simulink model "DAS"  (R2012b)
settings: Solver=FixedStepDiscrete  StartTime=0.0  StopTime=inf  FixedStep=0.1  RelTol=1e-3
PreLoadFcn:
  | if exist('tl_preloadfcn','file'), tl_preloadfcn(gcs,101); end
PostLoadFcn:
  | if exist('tl_postloadfcn','file'), tl_postloadfcn(gcs,101); end
InitFcn:
  | if exist('tlds_init','file'), tlds_init(gcs); end
StartFcn:
  | if exist('tlds_start','file'), tlds_start(gcs); end
StopFcn:
  | if exist('tlds_stop','file'), tlds_stop(gcs); end
undefined symbols (not defined in the file): A, B, C, Dd, DEMO_FAS_Accusti_Threshold_Time, DEMO_FAS_BrakeBooster_Threshold, DEMO_FAS_CC_DELTA, DEMO_FAS_CC_Lvl2_Round, DEMO_FAS_CC_Min_Value, DEMO_FAS_Distance_Treshold_Far, DEMO_FAS_Distance_Treshold_Med, DEMO_FAS_Distance_Treshold_Near, DEMO_FAS_Distronic, DEMO_FAS_Emerg_Brake_Force1, DEMO_FAS_Emerg_Brake_Force2, DEMO_FAS_Emerg_Brake_Time1, DEMO_FAS_Emerg_Brake_Time2, DEMO_FAS_EmergencyBrake, DEMO_FAS_FollowToStop, DEMO_FAS_Limiter, DEMO_FAS_Limiter_DELTA, DEMO_FAS_Neg_Max_ms, DEMO_FAS_Opti_Threshold_Time, DEMO_FAS_Repeater, DEMO_FAS_Repeater_Time, DEMO_FAS_Signdetection, DEMO_FAS_Tempomat
(part 2 of 11)

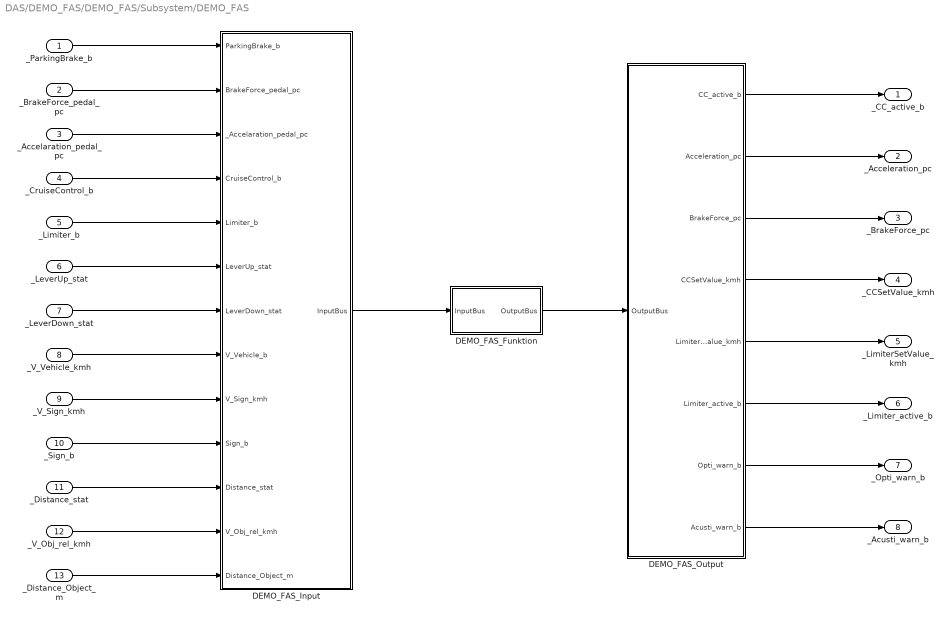
== system DAS/DEMO_FAS/DEMO_FAS/Subsystem/DEMO_FAS ==
  _ParkingBrake_b : Inport  PortDimensions=1  mask(TL_Inport){data={'output',{'variable','DEMO_FAS/i/Components/ParkingBrake_b'},'date',735342.43720311346}}
      settings: DeleteFcn=if exist('delete_tlblock','file')==2,delete_tlblock(gcbh);end  OpenFcn=if exist('tl_open_blockdlg','file')==2,tl_open_blockdlg(gcbh);else,open_system(gcbh,'parameter');end
      settings: CopyFcn=|
      | if exist('tl_reset_reviewflag','file')==2
      |     tl_reset_reviewflag(gcbh);
      | end
      | if exist('tl_check_ports','file')
      |     tl_check_ports(gcbh);
      | end
      settings: NameChangeFcn=|
      | if exist('rename_tlblock','file')==2,rename_tlblock(gcbh);end
      | if exist('tl_check_ports','file'), tl_check_ports(gcbh); end
      mask Help: eval(['if exist(''tl_online_help'',''file'') == 2, tl_online_help(''Topic'',''TL_Inport''),else, web([''jar:file:///'',matlabroot,''/help/toolbox/simulink/help.jar!/slref/' lower(get_param(gcbh,'Blocktype')) '.html''], ''-helpbrowser''),end'])
      mask Display: plot([0.2 0.35 NaN 0.65 0.8],[0 1 NaN 0 1]);
  _BrakeForce_pedal_pc : Inport  Port=2  PortDimensions=1  mask(TL_Inport){data={'output',{'variable','DEMO_FAS/i/Components/BrakeForce_pedal_pc'},'date',735342.4371075232}}
      settings: DeleteFcn=if exist('delete_tlblock','file')==2,delete_tlblock(gcbh);end  OpenFcn=if exist('tl_open_blockdlg','file')==2,tl_open_blockdlg(gcbh);else,open_system(gcbh,'parameter');end
      settings: CopyFcn=|
      | if exist('tl_reset_reviewflag','file')==2
      |     tl_reset_reviewflag(gcbh);
      | end
      | if exist('tl_check_ports','file')
      |     tl_check_ports(gcbh);
      | end
      settings: NameChangeFcn=|
      | if exist('rename_tlblock','file')==2,rename_tlblock(gcbh);end
      | if exist('tl_check_ports','file'), tl_check_ports(gcbh); end
      mask Help: eval(['if exist(''tl_online_help'',''file'') == 2, tl_online_help(''Topic'',''TL_Inport''),else, web([''jar:file:///'',matlabroot,''/help/toolbox/simulink/help.jar!/slref/' lower(get_param(gcbh,'Blocktype')) '.html''], ''-helpbrowser''),end'])
      mask Display: plot([0.2 0.35 NaN 0.65 0.8],[0 1 NaN 0 1]);
  _Accelaration_pedal_pc : Inport  Port=3  PortDimensions=1  mask(TL_Inport){data={'output',{'variable','DEMO_FAS/i/Components/Accelaration_pedal_pc'},'date',735342.43731296295}}
      settings: DeleteFcn=if exist('delete_tlblock','file')==2,delete_tlblock(gcbh);end  OpenFcn=if exist('tl_open_blockdlg','file')==2,tl_open_blockdlg(gcbh);else,open_system(gcbh,'parameter');end
      settings: CopyFcn=|
      | if exist('tl_reset_reviewflag','file')==2
      |     tl_reset_reviewflag(gcbh);
      | end
      | if exist('tl_check_ports','file')
      |     tl_check_ports(gcbh);
      | end
      settings: NameChangeFcn=|
      | if exist('rename_tlblock','file')==2,rename_tlblock(gcbh);end
      | if exist('tl_check_ports','file'), tl_check_ports(gcbh); end
      mask Help: eval(['if exist(''tl_online_help'',''file'') == 2, tl_online_help(''Topic'',''TL_Inport''),else, web([''jar:file:///'',matlabroot,''/help/toolbox/simulink/help.jar!/slref/' lower(get_param(gcbh,'Blocktype')) '.html''], ''-helpbrowser''),end'])
      mask Display: plot([0.2 0.35 NaN 0.65 0.8],[0 1 NaN 0 1]);
  _CruiseControl_b : Inport  Port=4  PortDimensions=1  mask(TL_Inport){data={'output',{'variable','DEMO_FAS/i/Components/CruiseControl_b'},'date',735342.43742563657}}
      settings: DeleteFcn=if exist('delete_tlblock','file')==2,delete_tlblock(gcbh);end  OpenFcn=if exist('tl_open_blockdlg','file')==2,tl_open_blockdlg(gcbh);else,open_system(gcbh,'parameter');end
      settings: CopyFcn=|
      | if exist('tl_reset_reviewflag','file')==2
      |     tl_reset_reviewflag(gcbh);
      | end
      | if exist('tl_check_ports','file')
      |     tl_check_ports(gcbh);
      | end
      settings: NameChangeFcn=|
      | if exist('rename_tlblock','file')==2,rename_tlblock(gcbh);end
      | if exist('tl_check_ports','file'), tl_check_ports(gcbh); end
      mask Help: eval(['if exist(''tl_online_help'',''file'') == 2, tl_online_help(''Topic'',''TL_Inport''),else, web([''jar:file:///'',matlabroot,''/help/toolbox/simulink/help.jar!/slref/' lower(get_param(gcbh,'Blocktype')) '.html''], ''-helpbrowser''),end'])
      mask Display: plot([0.2 0.35 NaN 0.65 0.8],[0 1 NaN 0 1]);
  _Limiter_b : Inport  Port=5  PortDimensions=1  mask(TL_Inport){data={'output',{'variable','DEMO_FAS/i/Components/Limiter_b'},'date',735342.4379789005}}
      settings: DeleteFcn=if exist('delete_tlblock','file')==2,delete_tlblock(gcbh);end  OpenFcn=if exist('tl_open_blockdlg','file')==2,tl_open_blockdlg(gcbh);else,open_system(gcbh,'parameter');end
      settings: CopyFcn=|
      | if exist('tl_reset_reviewflag','file')==2
      |     tl_reset_reviewflag(gcbh);
      | end
      | if exist('tl_check_ports','file')
      |     tl_check_ports(gcbh);
      | end
      settings: NameChangeFcn=|
      | if exist('rename_tlblock','file')==2,rename_tlblock(gcbh);end
      | if exist('tl_check_ports','file'), tl_check_ports(gcbh); end
      mask Help: eval(['if exist(''tl_online_help'',''file'') == 2, tl_online_help(''Topic'',''TL_Inport''),else, web([''jar:file:///'',matlabroot,''/help/toolbox/simulink/help.jar!/slref/' lower(get_param(gcbh,'Blocktype')) '.html''], ''-helpbrowser''),end'])
      mask Display: plot([0.2 0.35 NaN 0.65 0.8],[0 1 NaN 0 1]);
  _LeverUp_stat : Inport  Port=6  PortDimensions=1  mask(TL_Inport){data={'output',{'variable','DEMO_FAS/i/Components/LeverUp_stat'},'date',735382.56006785878}}
      settings: DeleteFcn=if exist('delete_tlblock','file')==2,delete_tlblock(gcbh);end  OpenFcn=if exist('tl_open_blockdlg','file')==2,tl_open_blockdlg(gcbh);else,open_system(gcbh,'parameter');end
      settings: CopyFcn=|
      | if exist('tl_reset_reviewflag','file')==2
      |     tl_reset_reviewflag(gcbh);
      | end
      | if exist('tl_check_ports','file')
      |     tl_check_ports(gcbh);
      | end
      settings: NameChangeFcn=|
      | if exist('rename_tlblock','file')==2,rename_tlblock(gcbh);end
      | if exist('tl_check_ports','file'), tl_check_ports(gcbh); end
      mask Help: eval(['if exist(''tl_online_help'',''file'') == 2, tl_online_help(''Topic'',''TL_Inport''),else, web([''jar:file:///'',matlabroot,''/help/toolbox/simulink/help.jar!/slref/' lower(get_param(gcbh,'Blocktype')) '.html''], ''-helpbrowser''),end'])
      mask Display: plot([0.2 0.35 NaN 0.65 0.8],[0 1 NaN 0 1]);
  _LeverDown_stat : Inport  Port=7  PortDimensions=1  mask(TL_Inport){data={'output',{'variable','DEMO_FAS/i/Components/LeverDown_stat'},'date',735382.55997754633}}
      settings: DeleteFcn=if exist('delete_tlblock','file')==2,delete_tlblock(gcbh);end  OpenFcn=if exist('tl_open_blockdlg','file')==2,tl_open_blockdlg(gcbh);else,open_system(gcbh,'parameter');end
      settings: CopyFcn=|
      | if exist('tl_reset_reviewflag','file')==2
      |     tl_reset_reviewflag(gcbh);
      | end
      | if exist('tl_check_ports','file')
      |     tl_check_ports(gcbh);
      | end
      settings: NameChangeFcn=|
      | if exist('rename_tlblock','file')==2,rename_tlblock(gcbh);end
      | if exist('tl_check_ports','file'), tl_check_ports(gcbh); end
      mask Help: eval(['if exist(''tl_online_help'',''file'') == 2, tl_online_help(''Topic'',''TL_Inport''),else, web([''jar:file:///'',matlabroot,''/help/toolbox/simulink/help.jar!/slref/' lower(get_param(gcbh,'Blocktype')) '.html''], ''-helpbrowser''),end'])
      mask Display: plot([0.2 0.35 NaN 0.65 0.8],[0 1 NaN 0 1]);
  _V_Vehicle_kmh : Inport  Port=8  PortDimensions=1  mask(TL_Inport){data={'output',{'variable','DEMO_FAS/i/Components/V_Vehicle_kmh'},'date',735342.43839186337}}
      settings: DeleteFcn=if exist('delete_tlblock','file')==2,delete_tlblock(gcbh);end  OpenFcn=if exist('tl_open_blockdlg','file')==2,tl_open_blockdlg(gcbh);else,open_system(gcbh,'parameter');end
      settings: CopyFcn=|
      | if exist('tl_reset_reviewflag','file')==2
      |     tl_reset_reviewflag(gcbh);
      | end
      | if exist('tl_check_ports','file')
      |     tl_check_ports(gcbh);
      | end
      settings: NameChangeFcn=|
      | if exist('rename_tlblock','file')==2,rename_tlblock(gcbh);end
      | if exist('tl_check_ports','file'), tl_check_ports(gcbh); end
      mask Help: eval(['if exist(''tl_online_help'',''file'') == 2, tl_online_help(''Topic'',''TL_Inport''),else, web([''jar:file:///'',matlabroot,''/help/toolbox/simulink/help.jar!/slref/' lower(get_param(gcbh,'Blocktype')) '.html''], ''-helpbrowser''),end'])
      mask Display: plot([0.2 0.35 NaN 0.65 0.8],[0 1 NaN 0 1]);
  _V_Sign_kmh : Inport  Port=9  PortDimensions=1  mask(TL_Inport){data={'output',{'variable','DEMO_FAS/i/Components/V_Sign_kmh'},'date',735382.5512869329}}
      settings: DeleteFcn=if exist('delete_tlblock','file')==2,delete_tlblock(gcbh);end  OpenFcn=if exist('tl_open_blockdlg','file')==2,tl_open_blockdlg(gcbh);else,open_system(gcbh,'parameter');end
      settings: CopyFcn=|
      | if exist('tl_reset_reviewflag','file')==2
      |     tl_reset_reviewflag(gcbh);
      | end
      | if exist('tl_check_ports','file')
      |     tl_check_ports(gcbh);
      | end
      settings: NameChangeFcn=|
      | if exist('rename_tlblock','file')==2,rename_tlblock(gcbh);end
      | if exist('tl_check_ports','file'), tl_check_ports(gcbh); end
      mask Help: eval(['if exist(''tl_online_help'',''file'') == 2, tl_online_help(''Topic'',''TL_Inport''),else, web([''jar:file:///'',matlabroot,''/help/toolbox/simulink/help.jar!/slref/' lower(get_param(gcbh,'Blocktype')) '.html''], ''-helpbrowser''),end'])
      mask Display: plot([0.2 0.35 NaN 0.65 0.8],[0 1 NaN 0 1]);
  _Sign_b : Inport  Port=10  PortDimensions=1  mask(TL_Inport){data={'output',{'variable','DEMO_FAS/i/Components/Sign_b'},'date',735382.5511889467}}
      settings: DeleteFcn=if exist('delete_tlblock','file')==2,delete_tlblock(gcbh);end  OpenFcn=if exist('tl_open_blockdlg','file')==2,tl_open_blockdlg(gcbh);else,open_system(gcbh,'parameter');end
      settings: CopyFcn=|
      | if exist('tl_reset_reviewflag','file')==2
      |     tl_reset_reviewflag(gcbh);
      | end
      | if exist('tl_check_ports','file')
      |     tl_check_ports(gcbh);
      | end
      settings: NameChangeFcn=|
      | if exist('rename_tlblock','file')==2,rename_tlblock(gcbh);end
      | if exist('tl_check_ports','file'), tl_check_ports(gcbh); end
      mask Help: eval(['if exist(''tl_online_help'',''file'') == 2, tl_online_help(''Topic'',''TL_Inport''),else, web([''jar:file:///'',matlabroot,''/help/toolbox/simulink/help.jar!/slref/' lower(get_param(gcbh,'Blocktype')) '.html''], ''-helpbrowser''),end'])
      mask Display: plot([0.2 0.35 NaN 0.65 0.8],[0 1 NaN 0 1]);
  _Distance_stat : Inport  Port=11  PortDimensions=1  mask(TL_Inport){data={'output',{'variable','DEMO_FAS/i/Components/Distance_stat'},'date',735382.55108829855}}
      settings: DeleteFcn=if exist('delete_tlblock','file')==2,delete_tlblock(gcbh);end  OpenFcn=if exist('tl_open_blockdlg','file')==2,tl_open_blockdlg(gcbh);else,open_system(gcbh,'parameter');end
      settings: CopyFcn=|
      | if exist('tl_reset_reviewflag','file')==2
      |     tl_reset_reviewflag(gcbh);
      | end
      | if exist('tl_check_ports','file')
      |     tl_check_ports(gcbh);
      | end
      settings: NameChangeFcn=|
      | if exist('rename_tlblock','file')==2,rename_tlblock(gcbh);end
      | if exist('tl_check_ports','file'), tl_check_ports(gcbh); end
      mask Help: eval(['if exist(''tl_online_help'',''file'') == 2, tl_online_help(''Topic'',''TL_Inport''),else, web([''jar:file:///'',matlabroot,''/help/toolbox/simulink/help.jar!/slref/' lower(get_param(gcbh,'Blocktype')) '.html''], ''-helpbrowser''),end'])
      mask Display: plot([0.2 0.35 NaN 0.65 0.8],[0 1 NaN 0 1]);
  _V_Obj_rel_kmh : Inport  Port=12  PortDimensions=1  mask(TL_Inport){data={'output',{'variable','DEMO_FAS/i/Components/V_Obj_rel_kmh'},'date',735382.55086876161}}
      settings: DeleteFcn=if exist('delete_tlblock','file')==2,delete_tlblock(gcbh);end  OpenFcn=if exist('tl_open_blockdlg','file')==2,tl_open_blockdlg(gcbh);else,open_system(gcbh,'parameter');end
      settings: CopyFcn=|
      | if exist('tl_reset_reviewflag','file')==2
      |     tl_reset_reviewflag(gcbh);
      | end
      | if exist('tl_check_ports','file')
      |     tl_check_ports(gcbh);
      | end
      settings: NameChangeFcn=|
      | if exist('rename_tlblock','file')==2,rename_tlblock(gcbh);end
      | if exist('tl_check_ports','file'), tl_check_ports(gcbh); end
      mask Help: eval(['if exist(''tl_online_help'',''file'') == 2, tl_online_help(''Topic'',''TL_Inport''),else, web([''jar:file:///'',matlabroot,''/help/toolbox/simulink/help.jar!/slref/' lower(get_param(gcbh,'Blocktype')) '.html''], ''-helpbrowser''),end'])
      mask Display: plot([0.2 0.35 NaN 0.65 0.8],[0 1 NaN 0 1]);
  _Distance_Object_m : Inport  Port=13  PortDimensions=1  mask(TL_Inport){data={'output',{'variable','DEMO_FAS/i/Components/Distance_Object_m'},'date',735382.55070593755}}
      settings: DeleteFcn=if exist('delete_tlblock','file')==2,delete_tlblock(gcbh);end  OpenFcn=if exist('tl_open_blockdlg','file')==2,tl_open_blockdlg(gcbh);else,open_system(gcbh,'parameter');end
      settings: CopyFcn=|
      | if exist('tl_reset_reviewflag','file')==2
      |     tl_reset_reviewflag(gcbh);
      | end
      | if exist('tl_check_ports','file')
      |     tl_check_ports(gcbh);
      | end
      settings: NameChangeFcn=|
      | if exist('rename_tlblock','file')==2,rename_tlblock(gcbh);end
      | if exist('tl_check_ports','file'), tl_check_ports(gcbh); end
      mask Help: eval(['if exist(''tl_online_help'',''file'') == 2, tl_online_help(''Topic'',''TL_Inport''),else, web([''jar:file:///'',matlabroot,''/help/toolbox/simulink/help.jar!/slref/' lower(get_param(gcbh,'Blocktype')) '.html''], ''-helpbrowser''),end'])
      mask Display: plot([0.2 0.35 NaN 0.65 0.8],[0 1 NaN 0 1]);
  DEMO_FAS_Funktion : Subsystem
  DEMO_FAS_Input : Subsystem
  DEMO_FAS_Output : Subsystem
  _CC_active_b : Outport  PortDimensions=1  mask(TL_Outport){data={'output',{'variable','DEMO_FAS/o/Components/CC_active_b'},'autosar',{'useautosarcommunication',1},'date',735441.38032703707}}
      settings: DeleteFcn=if exist('delete_tlblock','file')==2,delete_tlblock(gcbh);end  OpenFcn=if exist('tl_open_blockdlg','file')==2,tl_open_blockdlg(gcbh);else,open_system(gcbh,'parameter');end
      settings: CopyFcn=|
      | if exist('tl_reset_reviewflag','file')==2
      |     tl_reset_reviewflag(gcbh);
      | end
      | if exist('tl_check_ports','file')
      |     tl_check_ports(gcbh);
      | end
      settings: NameChangeFcn=|
      | if exist('rename_tlblock','file')==2,rename_tlblock(gcbh);end
      | if exist('tl_check_ports','file'), tl_check_ports(gcbh); end
      mask Help: eval(['if exist(''tl_online_help'',''file'') == 2, tl_online_help(''Topic'',''TL_Outport''),else, web([''jar:file:///'',matlabroot,''/help/toolbox/simulink/help.jar!/slref/' lower(get_param(gcbh,'Blocktype')) '.html''], ''-helpbrowser''),end'])
      mask Display: plot([0.2 0.35 NaN 0.65 0.8],[0 1 NaN 0 1]);
  _Acceleration_pc : Outport  Port=2  PortDimensions=1  mask(TL_Outport){data={'output',{'variable','DEMO_FAS/o/Components/Acceleration_pc'},'date',735346.41767621529}}
      settings: DeleteFcn=if exist('delete_tlblock','file')==2,delete_tlblock(gcbh);end  OpenFcn=if exist('tl_open_blockdlg','file')==2,tl_open_blockdlg(gcbh);else,open_system(gcbh,'parameter');end
      settings: CopyFcn=|
      | if exist('tl_reset_reviewflag','file')==2
      |     tl_reset_reviewflag(gcbh);
      | end
      | if exist('tl_check_ports','file')
      |     tl_check_ports(gcbh);
      | end
      settings: NameChangeFcn=|
      | if exist('rename_tlblock','file')==2,rename_tlblock(gcbh);end
      | if exist('tl_check_ports','file'), tl_check_ports(gcbh); end
      mask Help: eval(['if exist(''tl_online_help'',''file'') == 2, tl_online_help(''Topic'',''TL_Outport''),else, web([''jar:file:///'',matlabroot,''/help/toolbox/simulink/help.jar!/slref/' lower(get_param(gcbh,'Blocktype')) '.html''], ''-helpbrowser''),end'])
      mask Display: plot([0.2 0.35 NaN 0.65 0.8],[0 1 NaN 0 1]);
  _BrakeForce_pc : Outport  Port=3  PortDimensions=1  mask(TL_Outport){data={'output',{'variable','DEMO_FAS/o/Components/BrakeForce_pc'},'date',735360.45830094907}}
      settings: DeleteFcn=if exist('delete_tlblock','file')==2,delete_tlblock(gcbh);end  OpenFcn=if exist('tl_open_blockdlg','file')==2,tl_open_blockdlg(gcbh);else,open_system(gcbh,'parameter');end
      settings: CopyFcn=|
      | if exist('tl_reset_reviewflag','file')==2
      |     tl_reset_reviewflag(gcbh);
      | end
      | if exist('tl_check_ports','file')
      |     tl_check_ports(gcbh);
      | end
      settings: NameChangeFcn=|
      | if exist('rename_tlblock','file')==2,rename_tlblock(gcbh);end
      | if exist('tl_check_ports','file'), tl_check_ports(gcbh); end
      mask Help: eval(['if exist(''tl_online_help'',''file'') == 2, tl_online_help(''Topic'',''TL_Outport''),else, web([''jar:file:///'',matlabroot,''/help/toolbox/simulink/help.jar!/slref/' lower(get_param(gcbh,'Blocktype')) '.html''], ''-helpbrowser''),end'])
      mask Display: plot([0.2 0.35 NaN 0.65 0.8],[0 1 NaN 0 1]);
  _CCSetValue_kmh : Outport  Port=4  PortDimensions=1  mask(TL_Outport){data={'output',{'variable','DEMO_FAS/o/Components/CCSetValue_kmh'},'autosar',{'useautosarcommunication',1},'date',735346.41800862271}}
      settings: DeleteFcn=if exist('delete_tlblock','file')==2,delete_tlblock(gcbh);end  OpenFcn=if exist('tl_open_blockdlg','file')==2,tl_open_blockdlg(gcbh);else,open_system(gcbh,'parameter');end
      settings: CopyFcn=|
      | if exist('tl_reset_reviewflag','file')==2
      |     tl_reset_reviewflag(gcbh);
      | end
      | if exist('tl_check_ports','file')
      |     tl_check_ports(gcbh);
      | end
      settings: NameChangeFcn=|
      | if exist('rename_tlblock','file')==2,rename_tlblock(gcbh);end
      | if exist('tl_check_ports','file'), tl_check_ports(gcbh); end
      mask Help: eval(['if exist(''tl_online_help'',''file'') == 2, tl_online_help(''Topic'',''TL_Outport''),else, web([''jar:file:///'',matlabroot,''/help/toolbox/simulink/help.jar!/slref/' lower(get_param(gcbh,'Blocktype')) '.html''], ''-helpbrowser''),end'])
      mask Display: plot([0.2 0.35 NaN 0.65 0.8],[0 1 NaN 0 1]);
  _LimiterSetValue_kmh : Outport  Port=5  PortDimensions=1  mask(TL_Outport){data={'output',{'variable','DEMO_FAS/o/Components/LimiterSetValue_kmh'},'autosar',{'useautosarcommunication',1},'date',735346.41813160875}}
      settings: DeleteFcn=if exist('delete_tlblock','file')==2,delete_tlblock(gcbh);end  OpenFcn=if exist('tl_open_blockdlg','file')==2,tl_open_blockdlg(gcbh);else,open_system(gcbh,'parameter');end
      settings: CopyFcn=|
      | if exist('tl_reset_reviewflag','file')==2
      |     tl_reset_reviewflag(gcbh);
      | end
      | if exist('tl_check_ports','file')
      |     tl_check_ports(gcbh);
      | end
      settings: NameChangeFcn=|
      | if exist('rename_tlblock','file')==2,rename_tlblock(gcbh);end
      | if exist('tl_check_ports','file'), tl_check_ports(gcbh); end
      mask Help: eval(['if exist(''tl_online_help'',''file'') == 2, tl_online_help(''Topic'',''TL_Outport''),else, web([''jar:file:///'',matlabroot,''/help/toolbox/simulink/help.jar!/slref/' lower(get_param(gcbh,'Blocktype')) '.html''], ''-helpbrowser''),end'])
      mask Display: plot([0.2 0.35 NaN 0.65 0.8],[0 1 NaN 0 1]);
  _Limiter_active_b : Outport  Port=6  PortDimensions=1  mask(TL_Outport){data={'output',{'variable','DEMO_FAS/o/Components/Limiter_active_b'},'autosar',{'useautosarcommunication',1},'date',735441.38164214115}}
      settings: DeleteFcn=if exist('delete_tlblock','file')==2,delete_tlblock(gcbh);end  OpenFcn=if exist('tl_open_blockdlg','file')==2,tl_open_blockdlg(gcbh);else,open_system(gcbh,'parameter');end
      settings: CopyFcn=|
      | if exist('tl_reset_reviewflag','file')==2
      |     tl_reset_reviewflag(gcbh);
      | end
      | if exist('tl_check_ports','file')
      |     tl_check_ports(gcbh);
      | end
      settings: NameChangeFcn=|
      | if exist('rename_tlblock','file')==2,rename_tlblock(gcbh);end
      | if exist('tl_check_ports','file'), tl_check_ports(gcbh); end
      mask Help: eval(['if exist(''tl_online_help'',''file'') == 2, tl_online_help(''Topic'',''TL_Outport''),else, web([''jar:file:///'',matlabroot,''/help/toolbox/simulink/help.jar!/slref/' lower(get_param(gcbh,'Blocktype')) '.html''], ''-helpbrowser''),end'])
      mask Display: plot([0.2 0.35 NaN 0.65 0.8],[0 1 NaN 0 1]);
  _Opti_warn_b : Outport  Port=7  PortDimensions=1  mask(TL_Outport){data={'output',{'variable','DEMO_FAS/o/Components/Opti_warn_b'},'autosar',{'useautosarcommunication',1},'date',735382.56245105329}}
      settings: DeleteFcn=if exist('delete_tlblock','file')==2,delete_tlblock(gcbh);end  OpenFcn=if exist('tl_open_blockdlg','file')==2,tl_open_blockdlg(gcbh);else,open_system(gcbh,'parameter');end
      settings: CopyFcn=|
      | if exist('tl_reset_reviewflag','file')==2
      |     tl_reset_reviewflag(gcbh);
      | end
      | if exist('tl_check_ports','file')
      |     tl_check_ports(gcbh);
      | end
      settings: NameChangeFcn=|
      | if exist('rename_tlblock','file')==2,rename_tlblock(gcbh);end
      | if exist('tl_check_ports','file'), tl_check_ports(gcbh); end
      mask Help: eval(['if exist(''tl_online_help'',''file'') == 2, tl_online_help(''Topic'',''TL_Outport''),else, web([''jar:file:///'',matlabroot,''/help/toolbox/simulink/help.jar!/slref/' lower(get_param(gcbh,'Blocktype')) '.html''], ''-helpbrowser''),end'])
      mask Display: plot([0.2 0.35 NaN 0.65 0.8],[0 1 NaN 0 1]);
  _Acusti_warn_b : Outport  Port=8  PortDimensions=1  mask(TL_Outport){data={'output',{'variable','DEMO_FAS/o/Components/Acusti_warn_b'},'autosar',{'useautosarcommunication',1},'date',735382.56266055559}}
      settings: DeleteFcn=if exist('delete_tlblock','file')==2,delete_tlblock(gcbh);end  OpenFcn=if exist('tl_open_blockdlg','file')==2,tl_open_blockdlg(gcbh);else,open_system(gcbh,'parameter');end
      settings: CopyFcn=|
      | if exist('tl_reset_reviewflag','file')==2
      |     tl_reset_reviewflag(gcbh);
      | end
      | if exist('tl_check_ports','file')
      |     tl_check_ports(gcbh);
      | end
      settings: NameChangeFcn=|
      | if exist('rename_tlblock','file')==2,rename_tlblock(gcbh);end
      | if exist('tl_check_ports','file'), tl_check_ports(gcbh); end
      mask Help: eval(['if exist(''tl_online_help'',''file'') == 2, tl_online_help(''Topic'',''TL_Outport''),else, web([''jar:file:///'',matlabroot,''/help/toolbox/simulink/help.jar!/slref/' lower(get_param(gcbh,'Blocktype')) '.html''], ''-helpbrowser''),end'])
      mask Display: plot([0.2 0.35 NaN 0.65 0.8],[0 1 NaN 0 1]);
  wires:
  DEMO_FAS_Input/1(InputBus) -> DEMO_FAS_Funktion/1(InputBus)
  DEMO_FAS_Funktion/1(OutputBus) -> DEMO_FAS_Output/1(OutputBus)
  _V_Vehicle_kmh/1 -> DEMO_FAS_Input/8(V_Vehicle_b)
  _LeverDown_stat/1 -> DEMO_FAS_Input/7(LeverDown_stat)
  _LeverUp_stat/1 -> DEMO_FAS_Input/6(LeverUp_stat)
  _Limiter_b/1 -> DEMO_FAS_Input/5(Limiter_b)
  _Accelaration_pedal_pc/1 -> DEMO_FAS_Input/3(_Accelaration_pedal_pc)
  _CruiseControl_b/1 -> DEMO_FAS_Input/4(CruiseControl_b)
  _ParkingBrake_b/1 -> DEMO_FAS_Input/1(ParkingBrake_b)
  _BrakeForce_pedal_pc/1 -> DEMO_FAS_Input/2(BrakeForce_pedal_pc)
  DEMO_FAS_Output/2(Acceleration_pc) -> _Acceleration_pc/1
  DEMO_FAS_Output/1(CC_active_b) -> _CC_active_b/1
  DEMO_FAS_Output/4(CCSetValue_kmh) -> _CCSetValue_kmh/1
  DEMO_FAS_Output/5(LimiterSetValue_kmh) -> _LimiterSetValue_kmh/1
  DEMO_FAS_Output/6(Limiter_active_b) -> _Limiter_active_b/1
  DEMO_FAS_Output/3(BrakeForce_pc) -> _BrakeForce_pc/1
  _V_Sign_kmh/1 -> DEMO_FAS_Input/9(V_Sign_kmh)
  _Sign_b/1 -> DEMO_FAS_Input/10(Sign_b)
  _V_Obj_rel_kmh/1 -> DEMO_FAS_Input/12(V_Obj_rel_kmh)
  _Distance_Object_m/1 -> DEMO_FAS_Input/13(Distance_Object_m)
  _Distance_stat/1 -> DEMO_FAS_Input/11(Distance_stat)
  DEMO_FAS_Output/8(Acusti_warn_b) -> _Acusti_warn_b/1
  DEMO_FAS_Output/7(Opti_warn_b) -> _Opti_warn_b/1

== system DAS/Umgebung/Object/Accumulator_REL/Limit ==
  MX : Inport
  MN : Inport  Port=2
  u : Inport  Port=3
  LogOp_A : Logic
  LogOp_N : Logic  Operator=NOT  Inputs=1
  RelOp_MN : RelationalOperator  Operator=<  InputSameDT=on
  RelOp_MX : RelationalOperator  Operator=>  InputSameDT=on
  Switch_MN : Switch  Threshold=1  SaturateOnIntegerOverflow=on  InputSameDT=on
  Switch_MX : Switch  Threshold=1  SaturateOnIntegerOverflow=on  InputSameDT=on
  y : Outport  InitialOutput=0
  b_max : Outport  Port=2  InitialOutput=0
  b_min : Outport  Port=3  InitialOutput=0
  wires:
  Switch_MX/1 -> y/1
  u/1 -> RelOp_MN/1, RelOp_MX/1, Switch_MN/3
  RelOp_MN/1 -> Switch_MN/2, LogOp_A/2
  LogOp_A/1 -> b_min/1
  LogOp_N/1 -> LogOp_A/1
  Switch_MN/1 -> Switch_MX/3
  MN/1 -> Switch_MN/1, RelOp_MN/2
  MX/1 -> RelOp_MX/2, Switch_MX/1
  RelOp_MX/1 -> Switch_MX/2, LogOp_N/1, b_max/1

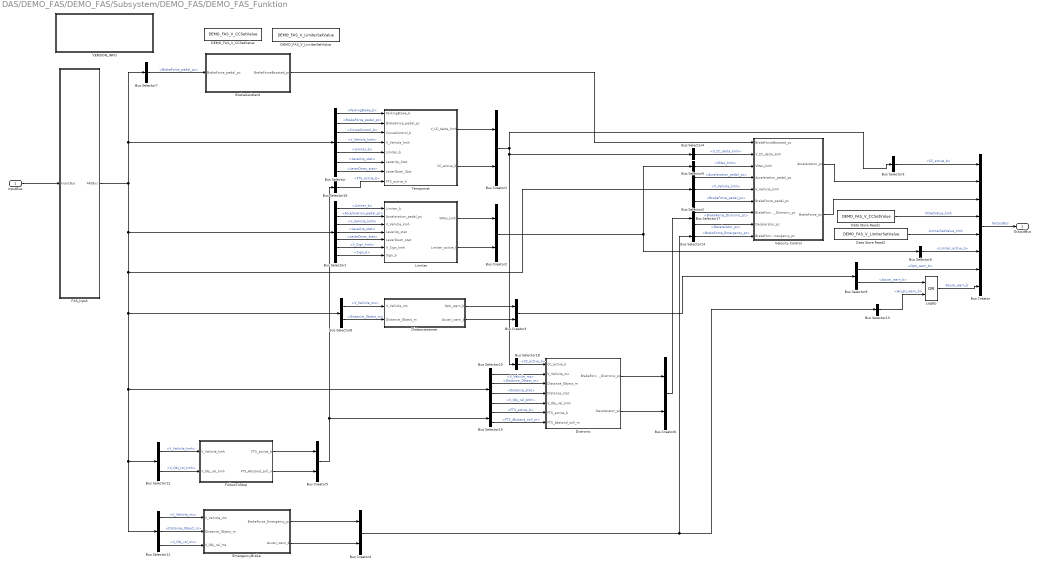
== system DAS/DEMO_FAS/DEMO_FAS/Subsystem/DEMO_FAS/DEMO_FAS_Funktion ==
  InputBus : Inport
  BrakeAssistant : Subsystem
  Bus Creator : BusCreator  Inputs=8
  Bus Creator{1..6} (6 alike) : BusCreator  Inputs=2
  Bus Selector : BusSelector  OutputSignals=ParkingBrake_b,BrakeForce_pedal_pc,CruiseControl_b,V_Vehicle_kmh,Limiter_b,LeverUp_stat,LeverDown_stat
  Bus Selector1 : BusSelector  OutputSignals=Limiter_b,Accelaration_pedal_pc,V_Vehicle_kmh,LeverUp_stat,LeverDown_stat,V_Sign_kmh,Sign_b
  Bus Selector10 : BusSelector  OutputSignals=V_Vehicle_ms,Distance_Object_m,Distance_stat,V_Obj_rel_kmh
  Bus Selector11 : BusSelector  OutputSignals=V_Vehicle_ms,Distance_Object_m,V_Obj_rel_ms
  Bus Selector12 : BusSelector  OutputSignals=V_Vehicle_kmh,V_Obj_rel_kmh
  Bus Selector13 : BusSelector  OutputSignals=Acusti_warn_b
  Bus Selector14 : BusSelector  OutputSignals=BrakeForce_Emergency_pc
  Bus Selector15 : BusSelector  OutputSignals=FTS_active_b,FTS_Abstand_soll_m
  Bus Selector16 : BusSelector  OutputSignals=FTS_active_b
  Bus Selector17 : BusSelector  OutputSignals=BrakeForce_Distronic_pc,Decelerator_pc
  Bus Selector18 : BusSelector  OutputSignals=CC_active_b
  Bus Selector2 : BusSelector  OutputSignals=Accelaration_pedal_pc,V_Vehicle_kmh,BrakeForce_pedal_pc
  Bus Selector3 : BusSelector  OutputSignals=CC_active_b
  Bus Selector4 : BusSelector  OutputSignals=V_CC_delta_kmh
  Bus Selector5 : BusSelector  OutputSignals=VMax_kmh
  Bus Selector6 : BusSelector  OutputSignals=Limiter_active_b
  Bus Selector7 : BusSelector  OutputSignals=BrakeForce_pedal_pc
  Bus Selector8 : BusSelector  OutputSignals=V_Vehicle_ms,Distance_Object_m
  Bus Selector9 : BusSelector  OutputSignals=Opti_warn_b,Acusti_warn_b
  DEMO_FAS_V_CCSetValue : DataStoreMemory  Description=|  DataStoreName=DEMO_FAS_V_CCSetValue  InitialValue=-1  mask(TL_DataStoreMemory){data={'output',{'variable','DEMO_FAS/en/Components/DEMO_FAS_V_CCSetValue'},'date',735343.64830100699}}
      | Data Store Memory block of dSPACE TargetLink.
      | Use this block to specify global variables within the production code application.
      settings: CopyFcn=if exist('tl_reset_reviewflag') == 2, tl_reset_reviewflag(gcbh); end  DeleteFcn=if exist('delete_tlblock','file')==2,delete_tlblock(gcbh);end  NameChangeFcn=if exist('rename_tlblock','file')==2,rename_tlblock(gcbh);end  OpenFcn=if exist('tl_open_blockdlg','file')==2,tl_open_blockdlg(gcbh);else,open_system(gcbh,'parameter');end
      mask Help: eval(['if exist(''tl_online_help'',''file'') == 2, tl_online_help(''Topic'',''TL_DataStoreMemory''),else, web([''jar:file:///'',matlabroot,''/help/toolbox/simulink/help.jar!/slref/' lower(get_param(gcbh,'Blocktype')) '.html''], ''-helpbrowser''),end'])
      mask Display: plot([-0.05, 1.05, NaN, -0.05, 1.05],[.01, .01, NaN, .99, .99])
  DEMO_FAS_V_LimiterSetValue : DataStoreMemory  Description=|  DataStoreName=DEMO_FAS_V_LimiterSetValue  mask(TL_DataStoreMemory){data={'output',{'variable','DEMO_FAS/en/Components/DEMO_FAS_V_LimiterSetValue'},'date',735342.52919987263}}
      | Data Store Memory block of dSPACE TargetLink.
      | Use this block to specify global variables within the production code application.
      settings: CopyFcn=if exist('tl_reset_reviewflag') == 2, tl_reset_reviewflag(gcbh); end  DeleteFcn=if exist('delete_tlblock','file')==2,delete_tlblock(gcbh);end  NameChangeFcn=if exist('rename_tlblock','file')==2,rename_tlblock(gcbh);end  OpenFcn=if exist('tl_open_blockdlg','file')==2,tl_open_blockdlg(gcbh);else,open_system(gcbh,'parameter');end
      mask Help: eval(['if exist(''tl_online_help'',''file'') == 2, tl_online_help(''Topic'',''TL_DataStoreMemory''),else, web([''jar:file:///'',matlabroot,''/help/toolbox/simulink/help.jar!/slref/' lower(get_param(gcbh,'Blocktype')) '.html''], ''-helpbrowser''),end'])
      mask Display: plot([-0.05, 1.05, NaN, -0.05, 1.05],[.01, .01, NaN, .99, .99])
  Data Store Read1 : DataStoreRead  Description=|  DataStoreName=DEMO_FAS_V_CCSetValue  mask(TL_DataStoreRead){data={'logdata',{'plotchannels',[]},'date',735342.58789737266}}
      | Data Store Read block of dSPACE TargetLink.
      | Use this block to specify inputs from global variables within the production code application.
      settings: DeleteFcn=if exist('delete_tlblock','file')==2,delete_tlblock(gcbh);end  NameChangeFcn=if exist('rename_tlblock','file')==2,rename_tlblock(gcbh);end  OpenFcn=if exist('tl_open_blockdlg','file')==2,tl_open_blockdlg(gcbh);else,open_system(gcbh,'parameter');end
      mask Help: eval(['if exist(''tl_online_help'',''file'') == 2, tl_online_help(''Topic'',''TL_DataStoreRead''),else, web([''jar:file:///'',matlabroot,''/help/toolbox/simulink/help.jar!/slref/' lower(get_param(gcbh,'Blocktype')) '.html''], ''-helpbrowser''),end'])
      mask Display: plot([-0.05, 1.05, NaN, -0.05, 1.05],[.01, .01, NaN, .99, .99])
  Data Store Read2 : DataStoreRead  Description=|  DataStoreName=DEMO_FAS_V_LimiterSetValue  mask(TL_DataStoreRead){data={'logdata',{'plotchannels',[]},'date',735342.52721385413}}
      | Data Store Read block of dSPACE TargetLink.
      | Use this block to specify inputs from global variables within the production code application.
      settings: DeleteFcn=if exist('delete_tlblock','file')==2,delete_tlblock(gcbh);end  NameChangeFcn=if exist('rename_tlblock','file')==2,rename_tlblock(gcbh);end  OpenFcn=if exist('tl_open_blockdlg','file')==2,tl_open_blockdlg(gcbh);else,open_system(gcbh,'parameter');end
      mask Help: eval(['if exist(''tl_online_help'',''file'') == 2, tl_online_help(''Topic'',''TL_DataStoreRead''),else, web([''jar:file:///'',matlabroot,''/help/toolbox/simulink/help.jar!/slref/' lower(get_param(gcbh,'Blocktype')) '.html''], ''-helpbrowser''),end'])
      mask Display: plot([-0.05, 1.05, NaN, -0.05, 1.05],[.01, .01, NaN, .99, .99])
  Distancewarner : Subsystem
  Distronic : Subsystem
  EmergencyBrake : Subsystem
  FAS_Input : Subsystem
  FollowToStop : Subsystem
  Limiter : Subsystem
  LogOp : Logic  Description=|  Operator=OR  AllPortsSameDT=off  mask(TL_LogicalOperator){data={'logdata',{'plotchannels',[]},'date',735383.53424436343}}
      | Logical operator block of dSPACE TargetLink.
      | 
      | The Logical Operator block performs any of these logical operations on its inputs: AND, OR, NAND, NOR, XOR, and NOT. A nonzero input is treated as TRUE (1), a zero input as FALSE (0). The output depends on the selected operator. The output is 1 if TRUE and 0 if FALSE.
      settings: DeleteFcn=if exist('delete_tlblock','file')==2,delete_tlblock(gcbh);end  NameChangeFcn=if exist('rename_tlblock','file')==2,rename_tlblock(gcbh);end  OpenFcn=if exist('tl_open_blockdlg','file')==2,tl_open_blockdlg(gcbh);else,open_system(gcbh,'parameter');end
      mask Help: eval(['if exist(''tl_online_help'',''file'') == 2, tl_online_help(''Topic'',''TL_LogicalOperator''),else, web([''jar:file:///'',matlabroot,''/help/toolbox/simulink/help.jar!/slref/' lower(get_param(gcbh,'Blocktype')) '.html''], ''-helpbrowser''),end'])
      mask Display: plot([-0.05, 1.05, NaN, -0.05, 1.05],[.01, .01, NaN, .99, .99])
  Tempomat : Subsystem
  VERSION_INFO : Subsystem  mask(VERSION_INFO_BLOCK){versinfo_data=struct('modname','DEMO_FAS/DEMO_FAS_Funktion','version','1.1.1','date','18-Apr-2013','author','YVEDUHR','modtype',3,'variant',0,'remark',{{'~'}},'copyright',['Daimler AG'],'SGMLdescr','','prefix','','pfx_act',0,'ntselect',3,'asize',0), versinfo_string=Model: DEMO_FAS/DEMO_FAS_Funktion\nVersion: 1.1.1\nDate: 18-Apr-2013\nAuthor: YVEDUHR\nModule: INTERNAL\n\nAll copyrights by Daimler AG}
      mask prompts: versinfo_data "Mask Parameter 1"; versinfo_string "Mask Parameter 2"
      mask help:
      | This is a Version Info Subsystem (empty)
      | All version Information is stored in Parameter "versinfo_data" and displayed
      settings: OpenFcn=edit_subsys_info('init')
      mask Display: disp(versinfo_string);
  Velocity Control : Subsystem
  OutputBus : Outport
  wires:
  InputBus/1 -> FAS_Input/1(InputBus)
  Bus Creator/1 -> OutputBus/1  "OutputBus"
  FAS_Input/1(FASBus) -> Bus Selector7/1, Bus Selector/1, Bus Selector11/1, Bus Selector12/1, Bus Selector10/1, Bus Selector8/1, Bus Selector2/1, Bus Selector1/1
  Bus Selector/1 -> Tempomat/1(ParkingBrake_b)  "<ParkingBrake_b>"
  Bus Selector/2 -> Tempomat/2(BrakeForce_pedal_pc)  "<BrakeForce_pedal_pc>"
  Bus Selector/6 -> Tempomat/6(LeverUp_Stat)  "<LeverUp_stat>"
  Bus Selector/7 -> Tempomat/7(LeverDown_Stat)  "<LeverDown_stat>"
  Bus Selector/4 -> Tempomat/4(V_Vehicle_kmh)  "<V_Vehicle_kmh>"
  Bus Selector/3 -> Tempomat/3(CruiseControl_b)  "<CruiseControl_b>"
  Bus Selector1/5 -> Limiter/5(LeverDown_stat)  "<LeverDown_stat>"
  Bus Selector1/1 -> Limiter/1(Limiter_b)  "<Limiter_b>"
  Bus Selector1/3 -> Limiter/3(V_Vehicle_kmh)  "<V_Vehicle_kmh>"
  Bus Selector1/4 -> Limiter/4(LeverUp_stat)  "<LeverUp_stat>"
  Bus Selector2/2 -> Velocity Control/5(V_Vehicle_kmh)  "<V_Vehicle_kmh>"
  Bus Selector2/1 -> Velocity Control/4(Accelaration_pedal_pc)  "<Accelaration_pedal_pc>"
  Velocity Control/1(Acceleration_pc) -> Bus Creator/2
  Bus Selector1/2 -> Limiter/2(Accelaration_pedal_pc)  "<Accelaration_pedal_pc>"
  Tempomat/1(V_CC_delta_kmh) -> Bus Creator1/1
  Tempomat/2(CC_active_b) -> Bus Creator1/2
  Bus Creator1/1 -> Bus Selector4/1, Bus Selector18/1, Bus Selector3/1
  Bus Selector3/1 -> Bus Creator/1  "<CC_active_b>"
  Bus Selector4/1 -> Velocity Control/2(V_CC_delta_kmh)  "<V_CC_delta_kmh>"
  Data Store Read1/1 -> Bus Creator/4  "CCSetValue_kmh"
  Data Store Read2/1 -> Bus Creator/5  "LimiterSetValue_kmh"
  Limiter/2(Limiter_active_b) -> Bus Creator2/2
  Limiter/1(VMax_kmh) -> Bus Creator2/1
  Bus Selector5/1 -> Velocity Control/3(VMax_kmh)  "<VMax_kmh>"
  Bus Creator2/1 -> Bus Selector5/1, Bus Selector6/1
  Bus Selector6/1 -> Bus Creator/6  "<Limiter_active_b>"
  Bus Selector/5 -> Tempomat/5(Limiter_b)  "<Limiter_b>"
  Bus Selector7/1 -> BrakeAssistant/1(BrakeForce_pedal_pc)  "<BrakeForce_pedal_pc>"
  BrakeAssistant/1(BrakeForceBoosted_pc) -> Velocity Control/1(BrakeForceBoosted_pc)
  Bus Selector2/3 -> Velocity Control/6(BrakeForce_pedal_pc)  "<BrakeForce_pedal_pc>"
  Velocity Control/2(BrakeForce_pc) -> Bus Creator/3
  Bus Selector1/7 -> Limiter/7(Sign_b)  "<Sign_b>"
  Bus Selector1/6 -> Limiter/6(V_Sign_kmh)  "<V_Sign_kmh>"
  Bus Selector8/1 -> Distancewarner/1(V_Vehicle_ms)  "<V_Vehicle_ms>"
  Bus Selector8/2 -> Distancewarner/2(Distance_Object_m)  "<Distance_Object_m>"
  Distancewarner/2(Acusti_warn_b) -> Bus Creator3/2
  Distancewarner/1(Opti_warn_b) -> Bus Creator3/1
  Bus Creator3/1 -> Bus Selector9/1
  Bus Selector9/1 -> Bus Creator/7  "<Opti_warn_b>"
  Bus Selector9/2 -> LogOp/1  "<Acusti_warn_b>"
  Bus Selector10/2 -> Distronic/3(Distance_Object_m)  "<Distance_Object_m>"
  Bus Selector10/1 -> Distronic/2(V_Vehicle_ms)  "<V_Vehicle_ms>"
  Bus Selector10/3 -> Distronic/4(Distance_stat)  "<Distance_stat>"
  Bus Selector10/4 -> Distronic/5(V_Obj_rel_kmh)  "<V_Obj_rel_kmh>"
  Distronic/1(BrakeForce_Distronic_pc) -> Bus Creator6/1
  Bus Selector11/2 -> EmergencyBrake/2(Distance_Object_m)  "<Distance_Object_m>"
  Bus Selector11/3 -> EmergencyBrake/3(V_Obj_rel_ms)  "<V_Obj_rel_ms>"
  Bus Selector11/1 -> EmergencyBrake/1(V_Vehicle_ms)  "<V_Vehicle_ms>"
  EmergencyBrake/1(BrakeForce_Emergency_pc) -> Bus Creator4/1
  EmergencyBrake/2(Acusti_warn_b) -> Bus Creator4/2
  LogOp/1 -> Bus Creator/8  "Acusti_warn_b"
  Bus Selector12/2 -> FollowToStop/2(V_Obj_rel_kmh)  "<V_Obj_rel_kmh>"
  Bus Selector12/1 -> FollowToStop/1(V_Vehicle_kmh)  "<V_Vehicle_kmh>"
  Bus Selector13/1 -> LogOp/2  "<Acusti_warn_b>"
  Bus Creator4/1 -> Bus Selector14/1, Bus Selector13/1
  Bus Selector14/1 -> Velocity Control/9(BrakeForce_Emergency_pc)  "<BrakeForce_Emergency_pc>"
  FollowToStop/1(FTS_active_b) -> Bus Creator5/1
  FollowToStop/2(FTS_Abstand_soll_m) -> Bus Creator5/2
  Bus Selector15/1 -> Distronic/6(FTS_active_b)  "<FTS_active_b>"
  Bus Selector16/1 -> Tempomat/8(FTS_active_b)  "<FTS_active_b>"
  Bus Creator5/1 -> Bus Selector16/1, Bus Selector15/1
  Bus Selector15/2 -> Distronic/7(FTS_Abstand_soll_m)  "<FTS_Abstand_soll_m>"
  Distronic/2(Decelerator_pc) -> Bus Creator6/2
  Bus Creator6/1 -> Bus Selector17/1
  Bus Selector17/2 -> Velocity Control/8(Decelerator_pc)  "<Decelerator_pc>"
  Bus Selector17/1 -> Velocity Control/7(BrakeForce_Distronic_pc)  "<BrakeForce_Distronic_pc>"
  Bus Selector18/1 -> Distronic/1(CC_active_b)  "<CC_active_b>"

== system DAS/DEMO_FAS/DEMO_FAS/Subsystem/DEMO_FAS/DEMO_FAS_Input ==
  ParkingBrake_b : Inport
  BrakeForce_pedal_pc : Inport  Port=2
  _Accelaration_pedal_pc : Inport  Port=3
  CruiseControl_b : Inport  Port=4
  Limiter_b : Inport  Port=5
  LeverUp_stat : Inport  Port=6
  LeverDown_stat : Inport  Port=7
  V_Vehicle_b : Inport  Port=8
  V_Sign_kmh : Inport  Port=9
  Sign_b : Inport  Port=10
  Distance_stat : Inport  Port=11
  V_Obj_rel_kmh : Inport  Port=12
  Distance_Object_m : Inport  Port=13
  Bus Creator : BusCreator  Inputs=13
  InputBus : Outport
  wires:
  LeverDown_stat/1 -> Bus Creator/7
  Limiter_b/1 -> Bus Creator/5
  BrakeForce_pedal_pc/1 -> Bus Creator/2
  CruiseControl_b/1 -> Bus Creator/4
  LeverUp_stat/1 -> Bus Creator/6
  ParkingBrake_b/1 -> Bus Creator/1
  Bus Creator/1 -> InputBus/1  "InputBus"
  V_Vehicle_b/1 -> Bus Creator/8
  _Accelaration_pedal_pc/1 -> Bus Creator/3
  V_Sign_kmh/1 -> Bus Creator/9
  Sign_b/1 -> Bus Creator/10
  V_Obj_rel_kmh/1 -> Bus Creator/12
  Distance_Object_m/1 -> Bus Creator/13
  Distance_stat/1 -> Bus Creator/11

== system DAS/DEMO_FAS/DEMO_FAS/Subsystem/DEMO_FAS/DEMO_FAS_Output ==
  OutputBus : Inport
  Bus Selector : BusSelector  OutputSignals=CC_active_b,Acceleration_pc,BrakeForce_pc,CCSetValue_kmh,LimiterSetValue_kmh,Limiter_active_b,Opti_warn_b,Acusti_warn_b
  CC_active_b : Outport
  Acceleration_pc : Outport  Port=2
  BrakeForce_pc : Outport  Port=3
  CCSetValue_kmh : Outport  Port=4
  LimiterSetValue_kmh : Outport  Port=5
  Limiter_active_b : Outport  Port=6
  Opti_warn_b : Outport  Port=7
  Acusti_warn_b : Outport  Port=8
  wires:
  OutputBus/1 -> Bus Selector/1
  Bus Selector/2 -> Acceleration_pc/1  "<Acceleration_pc>"
  Bus Selector/1 -> CC_active_b/1  "<CC_active_b>"
  Bus Selector/4 -> CCSetValue_kmh/1  "<CCSetValue_kmh>"
  Bus Selector/5 -> LimiterSetValue_kmh/1  "<LimiterSetValue_kmh>"
  Bus Selector/6 -> Limiter_active_b/1  "<Limiter_active_b>"
  Bus Selector/3 -> BrakeForce_pc/1  "<BrakeForce_pc>"
  Bus Selector/7 -> Opti_warn_b/1  "<Opti_warn_b>"
  Bus Selector/8 -> Acusti_warn_b/1  "<Acusti_warn_b>"

== system DAS/DEMO_FAS/DEMO_FAS/Subsystem/DEMO_FAS/DEMO_FAS_Funktion/BrakeAssistant ==
  BrakeForce_pedal_pc : Inport
  Brake_Booster : Subsystem  TreatAsAtomicUnit=on
  VERSION_INFO : Subsystem  mask(VERSION_INFO_BLOCK){versinfo_data=struct('modname','DEMO_FAS/DEMO_FAS_Funktion/BrakeAssistant','version','1.1.1','date','26-Apr-2013','author','YVEDUHR','modtype',3,'variant',0,'remark',{{'~'}},'copyright',['Daimler AG'],'SGMLdescr','','prefix','','pfx_act',0,'ntselect',3,'asize',0), versinfo_string=Model: DEMO_FAS/DEMO_FAS_Funktion/BrakeAssistant\nVersion: 1.1.1\nDate: 26-Apr-2013\nAuthor: YVEDUHR\nModule: INTERNAL\n\nAll copyrights by Daimler AG}
      mask prompts: versinfo_data "Mask Parameter 1"; versinfo_string "Mask Parameter 2"
      mask help:
      | This is a Version Info Subsystem (empty)
      | All version Information is stored in Parameter "versinfo_data" and displayed
      settings: OpenFcn=edit_subsys_info('init')
      mask Display: disp(versinfo_string);
  BrakeForceBoosted_pc : Outport
  wires:
  BrakeForce_pedal_pc/1 -> Brake_Booster/1(BrakeForce_pedal_pc)
  Brake_Booster/1(BrakeForceBoosted_pc) -> BrakeForceBoosted_pc/1

== system DAS/DEMO_FAS/DEMO_FAS/Subsystem/DEMO_FAS/DEMO_FAS_Funktion/Distancewarner ==
  V_Vehicle_ms : Inport
  Distance_Object_m : Inport  Port=2
  Distancewarner_Function : Subsystem  TreatAsAtomicUnit=on
  VERSION_INFO : Subsystem  mask(VERSION_INFO_BLOCK){versinfo_data=struct('modname','DEMO_FAS/DEMO_FAS_Funktion/Distancewarner','version','1.1.1','date','23-May-2013','author','YVEDUHR','modtype',3,'variant',0,'remark',{{'~'}},'copyright',['Daimler AG'],'SGMLdescr','','prefix','','pfx_act',0,'ntselect',3,'asize',0), versinfo_string=Model: DEMO_FAS/DEMO_FAS_Funktion/Distancewarner\nVersion: 1.1.1\nDate: 23-May-2013\nAuthor: YVEDUHR\nModule: INTERNAL\n\nAll copyrights by Daimler AG}
      mask prompts: versinfo_data "Mask Parameter 1"; versinfo_string "Mask Parameter 2"
      mask help:
      | This is a Version Info Subsystem (empty)
      | All version Information is stored in Parameter "versinfo_data" and displayed
      settings: OpenFcn=edit_subsys_info('init')
      mask Display: disp(versinfo_string);
  Opti_warn_b : Outport
  Acusti_warn_b : Outport  Port=2  InitialOutput=0
  wires:
  Distancewarner_Function/1(Opti_warn_b) -> Opti_warn_b/1
  Distancewarner_Function/2(Acusti_warn_b) -> Acusti_warn_b/1
  V_Vehicle_ms/1 -> Distancewarner_Function/1(V_Vehicle_ms)
  Distance_Object_m/1 -> Distancewarner_Function/2(Distance_Object_m)

== system DAS/DEMO_FAS/DEMO_FAS/Subsystem/DEMO_FAS/DEMO_FAS_Funktion/Distronic ==
  CC_active_b : Inport
  V_Vehicle_ms : Inport  Port=2
  Distance_Object_m : Inport  Port=3
  Distance_stat : Inport  Port=4
  V_Obj_rel_kmh : Inport  Port=5
  FTS_active_b : Inport  Port=6
  FTS_Abstand_soll_m : Inport  Port=7
  Bus Creator{1..4} (4 alike) : BusCreator  Inputs=2
  Bus Selector : BusSelector  OutputSignals=BrakeForce_Distronic_pc,Decelerator_pc
  DEMO_FAS_Distronic : Constant  Description=|  Value=DEMO_FAS_Distronic  SampleTime=-1  mask(TL_Constant){data={'output',{'variable','DEMO_FAS/p/Components/DEMO_FAS_Distronic'},'date',735382.58604282408}}
      | Constant block of dSPACE TargetLink.
      | 
      | Output signal keeps the given constant value.
      settings: DeleteFcn=if exist('delete_tlblock','file')==2,delete_tlblock(gcbh);end  NameChangeFcn=if exist('rename_tlblock','file')==2,rename_tlblock(gcbh);end  OpenFcn=if exist('tl_open_blockdlg','file')==2,tl_open_blockdlg(gcbh);else,open_system(gcbh,'parameter');end
      mask Help: eval(['if exist(''tl_online_help'',''file'') == 2, tl_online_help(''Topic'',''TL_Constant''),else, web([''jar:file:///'',matlabroot,''/help/toolbox/simulink/help.jar!/slref/' lower(get_param(gcbh,'Blocktype')) '.html''], ''-helpbrowser''),end'])
      mask Display: plot([-0.05, 1.05, NaN, -0.05, 1.05],[.01, .01, NaN, .99, .99])
  Distronic_Deactive : Subsystem  TreatAsAtomicUnit=on
  Distronic_Disabled : Subsystem  TreatAsAtomicUnit=on
  Distronic_Enabled : Subsystem
  Distronic_FTS_Enabled : Subsystem
  If : If  NumInputs=3  IfExpression=u1 & u2 & ~u3  ElseIfExpressions=u1 & u2 & u3 ,u1 & ~u2
  Merge : Merge  Description=|  Inputs=4  mask(TL_Merge){data={'date',735389.38576818292}}
      | Merge block of dSPACE TargetLink.
      | 
      | Use this block instead of Simulink's Merge block if you wish to control how merge variables should be generated.
      settings: CopyFcn=if exist('tl_reset_reviewflag') == 2, tl_reset_reviewflag(gcbh); end  DeleteFcn=if exist('delete_tlblock','file')==2,delete_tlblock(gcbh);end  NameChangeFcn=if exist('rename_tlblock','file')==2,rename_tlblock(gcbh);end  OpenFcn=if exist('tl_open_blockdlg','file')==2,tl_open_blockdlg(gcbh);else,open_system(gcbh,'parameter');end
      mask Help: eval(['if exist(''tl_online_help'',''file'') == 2, tl_online_help(''Topic'',''TL_Merge''),else, web([''jar:file:///'',matlabroot,''/help/toolbox/simulink/help.jar!/slref/' lower(get_param(gcbh,'Blocktype')) '.html''], ''-helpbrowser''),end'])
      mask Display: plot([-0.05, 1.05, NaN, -0.05, 1.05],[.01, .01, NaN, .99, .99])
  VERSION_INFO : Subsystem  mask(VERSION_INFO_BLOCK){versinfo_data=struct('modname','DEMO_FAS/DEMO_FAS_Funktion/Distronic','version','1.1.1','date','28-May-2013','author','YVEDUHR','modtype',3,'variant',0,'remark',{{'~'}},'copyright',['Daimler AG'],'SGMLdescr','','prefix','','pfx_act',0,'ntselect',3,'asize',0), versinfo_string=Model: DEMO_FAS/DEMO_FAS_Funktion/Distronic\nVersion: 1.1.1\nDate: 28-May-2013\nAuthor: YVEDUHR\nModule: INTERNAL\n\nAll copyrights by Daimler AG}
      mask prompts: versinfo_data "Mask Parameter 1"; versinfo_string "Mask Parameter 2"
      mask help:
      | This is a Version Info Subsystem (empty)
      | All version Information is stored in Parameter "versinfo_data" and displayed
      settings: OpenFcn=edit_subsys_info('init')
      mask Display: disp(versinfo_string);
  BrakeForce_Distronic_pc : Outport
  Decelerator_pc : Outport  Port=2  OutputWhenDisabled=reset  InitialOutput=0
  wires:
  DEMO_FAS_Distronic/1 -> If/1
  CC_active_b/1 -> If/2
  Distance_Object_m/1 -> Distronic_FTS_Enabled/1(Distance_Object_m), Distronic_Enabled/2(Distance_Object_m)
  V_Obj_rel_kmh/1 -> Distronic_FTS_Enabled/3(V_Obj_rel_kmh), Distronic_Enabled/4(V_Obj_rel_kmh)
  V_Vehicle_ms/1 -> Distronic_Enabled/1(V_Vehicle_ms)
  Distance_stat/1 -> Distronic_Enabled/3(Distance_stat)
  If/1 -> Distronic_Enabled/Action
  If/2 -> Distronic_FTS_Enabled/Action
  If/4 -> Distronic_Deactive/Action
  Bus Selector/1 -> BrakeForce_Distronic_pc/1  "<BrakeForce_Distronic_pc>"
  FTS_active_b/1 -> If/3
  If/3 -> Distronic_Disabled/Action
  FTS_Abstand_soll_m/1 -> Distronic_FTS_Enabled/2(FTS_Abstand_soll_m)
  Distronic_Enabled/1(BrakeForce_Distronic_pc) -> Bus Creator1/1
  Bus Creator1/1 -> Merge/1
  Distronic_Enabled/2(Decelerator_pc) -> Bus Creator1/2
  Distronic_Disabled/1(BrakeForce_Distronic_pc) -> Bus Creator2/1
  Distronic_Disabled/2(Decelerator_pc) -> Bus Creator2/2
  Bus Creator2/1 -> Merge/3
  Bus Creator3/1 -> Merge/4
  Distronic_Deactive/1(BrakeForce_Distronic_pc) -> Bus Creator3/1
  Distronic_Deactive/2(Decelerator_pc) -> Bus Creator3/2
  Merge/1 -> Bus Selector/1  "BrakeForce_Distronic_pc"
  Bus Creator4/1 -> Merge/2
  Distronic_FTS_Enabled/1(BrakeForce_Distronic_pc) -> Bus Creator4/1
  Distronic_FTS_Enabled/2(Decelerator_pc) -> Bus Creator4/2
  Bus Selector/2 -> Decelerator_pc/1  "<Decelerator_pc>"
